simulink model "single_phase_converter_dq_i_pi_closeloop"  (R2022b)
settings: Solver=VariableStepAuto  StartTime=0.0  StopTime=0.1  FixedStep=1e-6  MaxStep=1e-8  RelTol=1e-7
model workspace (MAT data in the model file):
  Ts = 2.5e-05
  wr = 314.159265359
libraries: spsMosfetLib x4, spsSeriesRLCBranchLib x4, slpidlib x2, spsCurrentMeasurementLib x1, spsDCVoltageSourceLib x1, spsIdealSwitchLib x1, simulink x1, dspsigops x1, sps_lib x1
settings Model: Creator=SSC  LastModifiedBy=SSC

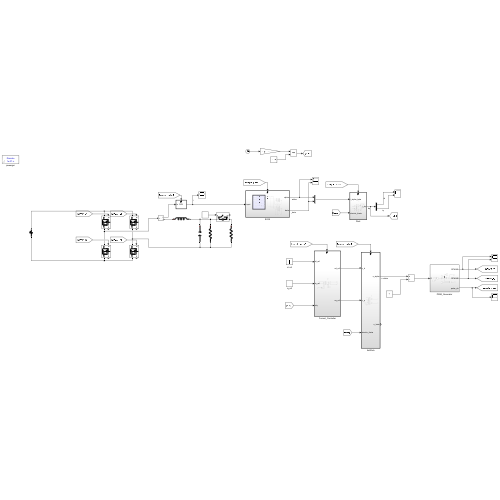
[thumbnail: Simulink's stored preview of the top-level diagram]
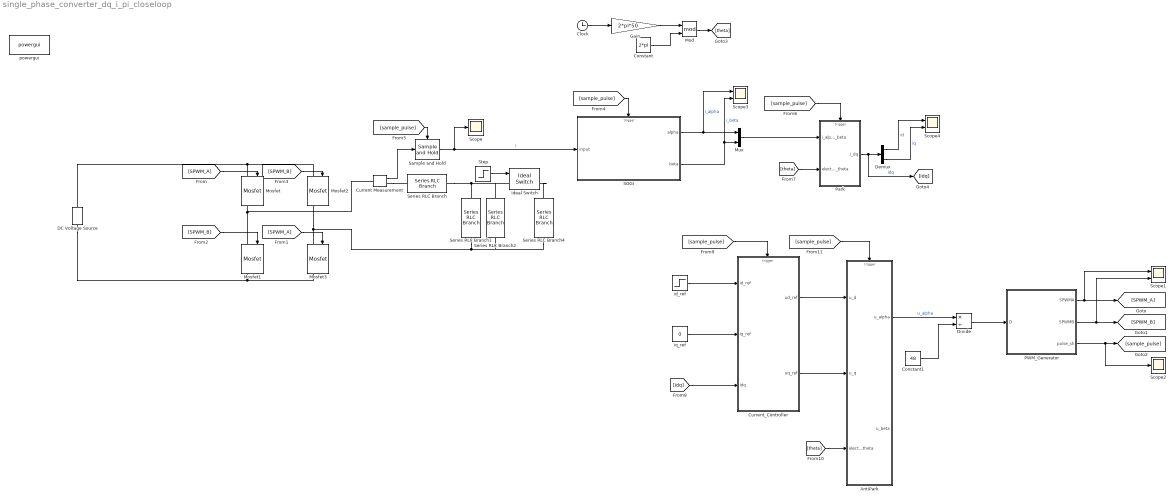
== system single_phase_converter_dq_i_pi_closeloop ==
  AntiPark : Subsystem
  Clock : Clock
  Constant : Constant  Value=2*pi
  Constant1 : Constant  Value=48
  Current Measurement : spsCurrentMeasurementLib/Current Measurement  PhasorSimulation=off  OutputType=Complex  PSBequivalent=0
  Current_Controller : Subsystem
  DC Voltage Source : spsDCVoltageSourceLib/DC Voltage Source  Amplitude=48  Measurements=None
  Demux : Demux  Outputs=2
  Divide : Product  Inputs=*/
  Gain : Gain  Gain=2*pi*50
  Ideal Switch : spsIdealSwitchLib/Ideal Switch  Ron=1e-5  Lon=0  IC=0  Rs=1e5  Cs=inf  Measurements=on
  Mod : Math  Operator=mod
  Mosfet{,1..3} (4 alike) : spsMosfetLib/Mosfet  Ron=0.1  Lon=0  Rd=0.01  Vfd=0  IC=0  Rs=1e5  Cs=inf  Measurements=on
  Mux : Mux  Inputs=2
  PWM_Generator : Subsystem
  Park : Subsystem
  SOGI : Subsystem  TreatAsAtomicUnit=on
  Sample and Hold : dspsigops/Sample and Hold  trig=Rising edge  initCond=0  latchinput=off
  Scope : Scope
  Scope1 : Scope  NumInputPorts=2
  Scope2 : Scope
  Scope3 : Scope  NumInputPorts=2
  Scope4 : Scope  NumInputPorts=2
  Series RLC Branch : spsSeriesRLCBranchLib/Series RLC Branch  LConnTagsString=__new0  RConnTagsString=__new0  BranchType=L  Resistance=1  Inductance=2e-3  SetiL0=off  InitialCurrent=0  Capacitance=1e-6  Setx0=off  InitialVoltage=0  Measurements=None
  Series RLC Branch1 : spsSeriesRLCBranchLib/Series RLC Branch  LConnTagsString=__new0  RConnTagsString=__new0  BranchType=C  Resistance=1  Inductance=1e-3  SetiL0=off  InitialCurrent=0  Capacitance=25e-6  Setx0=off  InitialVoltage=0  Measurements=None
  Series RLC Branch2 : spsSeriesRLCBranchLib/Series RLC Branch  LConnTagsString=__new0  RConnTagsString=__new0  BranchType=R  Resistance=12  Inductance=1e-3  SetiL0=off  InitialCurrent=0  Capacitance=1e-6  Setx0=off  InitialVoltage=0  Measurements=None
  Series RLC Branch4 : spsSeriesRLCBranchLib/Series RLC Branch  LConnTagsString=__new0  RConnTagsString=__new0  BranchType=R  Resistance=12  Inductance=1e-3  SetiL0=off  InitialCurrent=0  Capacitance=1e-6  Setx0=off  InitialVoltage=0  Measurements=None
  Step : Step  Time=0.1  SampleTime=0
  id_ref : Step  Time=0.05  Before=2  SampleTime=0
  iq_ref : Constant  Value=0
  powergui : sps_lib/powergui  Priority=1  SimulationMode=Discrete  SampleTime=1e-7  frequency=60  Iterations=50  frequencyindice=0  Pbase=100e6  ErrMax=1e-4  UnitsV=kV  UnitsW=MW  buscounter=0  FunctionMessages=off  echomessages=off  EnableUseOfTLC=off  CurrentSourceSwitches=off  DisableSnubberDevices=off  DisableRonSwitches=off  DisableVfSwitches=off  DisplayEquations=off  AutomaticDiscreteSolvers=off  SolverType=Tustin/Backward Euler (TBE)  Interpol=off  ExternalGateDelay=off  methode=off  Ts=100  x0status=blocks  SPID=on  SwTol=0  HookPort=off  NonlinearTolerance=1e-4  nMaxIteration=100  ContinueOnMaxIteration=off  RestoreLinks=warning  ResistiveCurrentMeasurement=off  Frange=[0:2:500]  Ylog=off  Xlog=on  ShowGrid=off  save=off  variable=ZData  structure=0  ZoomFFT=off  StartTime=0.0  cycles=1  DisplayStyle=1  fundamental=60  FreqAxis=off  MaxFrequency=1000  frequencyindicesteady=1  RmsSteady=1  display=off
  wires:
  Sample and Hold/1 -> SOGI/1(input), Scope/1  "i"
  [SPWM_A] -> Mosfet/1
  [SPWM_A] -> Mosfet3/1
  [SPWM_B] -> Mosfet1/1
  [SPWM_B] -> Mosfet2/1
  PWM_Generator/1(SPWMA) -> [SPWM_A], Scope1/1
  PWM_Generator/2(SPWMB) -> [SPWM_B], Scope1/2
  Divide/1 -> PWM_Generator/1(D)
  PWM_Generator/3(pulse_sh) -> Scope2/1, [sample_pulse]
  [sample_pulse] -> SOGI/Trigger
  Step/1 -> Ideal Switch/1
  Current Measurement/1 -> Sample and Hold/1
  [sample_pulse] -> Sample and Hold/Trigger
  SOGI/1(alpha) -> Mux/1, Scope3/1  "i_alpha"
  SOGI/2(beta) -> Mux/2, Scope3/2  "i_beta"
  Clock/1 -> Gain/1
  Gain/1 -> Mod/1
  Constant/1 -> Mod/2
  Mod/1 -> [theta]
  Mux/1 -> Park/1(i_alpha_beta)
  [sample_pulse] -> Park/Trigger
  [theta] -> Park/2(electric_theta)
  Park/1(i_dq) -> [idq], Demux/1  "idq"
  Demux/1 -> Scope4/1  "id"
  Demux/2 -> Scope4/2  "iq"
  iq_ref/1 -> Current_Controller/2(iq_ref)
  [idq] -> Current_Controller/3(idq)
  [sample_pulse] -> Current_Controller/Trigger
  Current_Controller/1(ud_ref) -> AntiPark/1(u_d)
  Current_Controller/2(uq_ref) -> AntiPark/2(u_q)
  [theta] -> AntiPark/3(electric_theta)
  [sample_pulse] -> AntiPark/Trigger
  AntiPark/1(u_alpha) -> Divide/1  "u_alpha"
  Constant1/1 -> Divide/2
  id_ref/1 -> Current_Controller/1(id_ref)
  connections:
  Series RLC Branch/RConn1 -- Series RLC Branch2/LConn1 -- Ideal Switch/LConn1 -- Series RLC Branch1/LConn1
  Mosfet1/LConn1 -- Current Measurement/LConn1 -- Mosfet/RConn1
  Mosfet/LConn1 -- Mosfet2/LConn1 -- DC Voltage Source/RConn1
  DC Voltage Source/LConn1 -- Mosfet3/RConn1 -- Mosfet1/RConn1
  Mosfet3/LConn1 -- Mosfet2/RConn1 -- Series RLC Branch2/RConn1 -- Series RLC Branch4/RConn1 -- Series RLC Branch1/RConn1
  Ideal Switch/RConn1 -- Series RLC Branch4/LConn1
  Current Measurement/RConn1 -- Series RLC Branch/LConn1

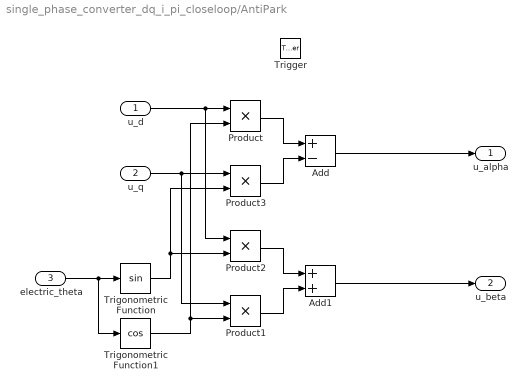
== system single_phase_converter_dq_i_pi_closeloop/AntiPark ==
  u_d : Inport
  u_q : Inport  Port=2
  electric_theta : Inport  Port=3
  Trigger : TriggerPort  VariantControl=(inherit)
  Add : Sum  Inputs=+-
  Add1 : Sum
  Product{,1..3} (4 alike) : Product
  Trigonometric Function : Trigonometry
  Trigonometric Function1 : Trigonometry  Operator=cos
  u_alpha : Outport
  u_beta : Outport  Port=2
  wires:
  electric_theta/1 -> Trigonometric Function1/1, Trigonometric Function/1
  u_d/1 -> Product2/1, Product/1
  Trigonometric Function1/1 -> Product/2, Product1/2
  u_q/1 -> Product1/1, Product3/1
  Trigonometric Function/1 -> Product2/2, Product3/2
  Product/1 -> Add/1
  Product3/1 -> Add/2
  Add/1 -> u_alpha/1
  Product2/1 -> Add1/1
  Product1/1 -> Add1/2
  Add1/1 -> u_beta/1

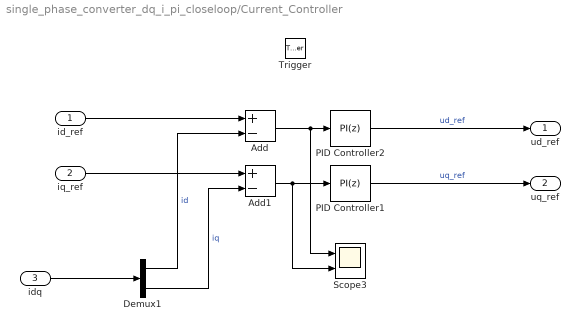
== system single_phase_converter_dq_i_pi_closeloop/Current_Controller ==
  id_ref : Inport
  iq_ref : Inport  Port=2
  idq : Inport  Port=3
  Trigger : TriggerPort  VariantControl=(inherit)
  Add : Sum  Inputs=+-
  Add1 : Sum  Inputs=+-
  Demux1 : Demux  Outputs=2
  PID Controller1 : slpidlib/PID Controller  Controller=PI  Form=Parallel  TimeDomain=Discrete-time  UseExternalTs=off  SampleTime=-1  IntegratorMethod=Trapezoidal  FilterMethod=Forward Euler  ControllerParametersSource=internal  P=1  I=1000  UseKiTs=off  D=0  N=100  UseFilter=on  TunerSelectOption=Transfer Function Based (PID Tuner App)  InitialConditionSource=internal  InitialConditionForIntegrator=0  InitialConditionForFilter=0  DifferentiatorICPrevScaledInput=0  ExternalReset=none  TrackingMode=off  Kt=1  LimitOutput=off  SatLimitsSource=internal  UpperSaturationLimit=inf  LowerSaturationLimit=-inf  LinearizeAsGain=on  AntiWindupMode=none  Kb=1  LimitIntegrator=off  UpperIntegratorSaturationLimit=inf  LowerIntegratorSaturationLimit=-inf  POutMin=[]  POutMax=[]  IOutMin=[]  IOutMax=[]  DOutMin=[]  DOutMax=[]  NOutMin=[]  NOutMax=[]  SumOutMin=[]  SumOutMax=[]  SaturationOutMin=[]  SaturationOutMax=[]  PParamMin=[]  PParamMax=[]  IParamMin=[]  IParamMax=[]  DParamMin=[]  DParamMax=[]  NParamMin=[]  NParamMax=[]  KbParamMin=[]  KbParamMax=[]  KtParamMin=[]  KtParamMax=[]  KbOutMin=[]  KbOutMax=[]  KtOutMin=[]  KtOutMax=[]  IntegratorOutMin=[]  IntegratorOutMax=[]  FilterOutMin=[]  FilterOutMax=[]  SumI1OutMin=[]  SumI1OutMax=[]  SumI2OutMin=[]  SumI2OutMax=[]  SumI3OutMin=[]  SumI3OutMax=[]  SumI4OutMin=[]  SumI4OutMax=[]  SumDOutMin=[]  SumDOutMax=[]  DifferentiatorOutMin=[]  DifferentiatorOutMax=[]  FilterDiffOutCoefMin=[]  FilterDiffOutCoefMax=[]  ReciprocalOutMin=[]  ReciprocalOutMax=[]  SumDenOutMin=[]  SumDenOutMax=[]  SumNumOutMin=[]  SumNumOutMax=[]  DivideOutMin=[]  DivideOutMax=[]  UdiffTsProdOutMin=[]  UdiffTsProdOutMax=[]  NTsProdOutMin=[]  NTsProdOutMax=[]  UintegralTsProdOutMin=[]  UintegralTsProdOutMax=[]  UngainTsProdOutMin=[]  UngainTsProdOutMax=[]  ClampingZeroOutDataTypeStr=Inherit: Inherit via back propagation  ClampingZeroOutMin=[]  ClampingZeroOutMax=[]  FilterDenConstantOutDataTypeStr=Inherit: Inherit via back propagation  FilterDenConstantOutMin=[]  FilterDenConstantOutMax=[]  PCopyOutDataTypeStr=Inherit: Inherit via back propagation  PCopyOutMin=[]  PCopyOutMax=[]  NCopyOutDataTypeStr=Inherit: Inherit via back propagation  NCopyOutMin=[]  NCopyOutMax=[]  IntegratorContinuousStateAttributes=''  IntegratorStateMustResolveToSignalObject=off  IntegratorRTWStateStorageClass=Auto  FilterContinuousStateAttributes=''  FilterStateMustResolveToSignalObject=off  FilterRTWStateStorageClass=Auto  ParallelPVariant=InternalParameters  IdealPVariant=Disabled  IVariant=InternalParameters  DVariant=Disabled  IntegratorVariant=Discrete  SatVariant=Disabled  AWVariant=Passthrough  PCopyVariant=Disabled  TRVariant=Disabled  FdbkBlocksVariant=Forward  IdealPFdbkVariant=Disabled  SatFdbkVariant=Disabled  DerivativeFilterVariant=Disabled  NVariant=Disabled  NCopyVariant=Disabled_SignalSpec  FilterICVariant=Disabled  IntegratorICVariant=InternalICs  ExternalResetVariant=Disabled  TRSumVariant=Passthrough  SumFdbkVariant=Disabled  SumVariant=Sum_PI  TsampFilterVariant=InternalTs  TsampNgainVariant=Passthrough  TsampIntegralVariant=Passthrough  ExternalSaturationOutDataTypeStr=Inherit: Same as second input
  PID Controller2 : slpidlib/PID Controller  Controller=PI  Form=Parallel  TimeDomain=Discrete-time  UseExternalTs=off  SampleTime=-1  IntegratorMethod=Trapezoidal  FilterMethod=Forward Euler  ControllerParametersSource=internal  P=10  I=1000  UseKiTs=off  D=0  N=100  UseFilter=on  TunerSelectOption=Transfer Function Based (PID Tuner App)  InitialConditionSource=internal  InitialConditionForIntegrator=0  InitialConditionForFilter=0  DifferentiatorICPrevScaledInput=0  ExternalReset=none  TrackingMode=off  Kt=1  LimitOutput=off  SatLimitsSource=internal  UpperSaturationLimit=inf  LowerSaturationLimit=-inf  LinearizeAsGain=on  AntiWindupMode=none  Kb=1  LimitIntegrator=off  UpperIntegratorSaturationLimit=inf  LowerIntegratorSaturationLimit=-inf  POutMin=[]  POutMax=[]  IOutMin=[]  IOutMax=[]  DOutMin=[]  DOutMax=[]  NOutMin=[]  NOutMax=[]  SumOutMin=[]  SumOutMax=[]  SaturationOutMin=[]  SaturationOutMax=[]  PParamMin=[]  PParamMax=[]  IParamMin=[]  IParamMax=[]  DParamMin=[]  DParamMax=[]  NParamMin=[]  NParamMax=[]  KbParamMin=[]  KbParamMax=[]  KtParamMin=[]  KtParamMax=[]  KbOutMin=[]  KbOutMax=[]  KtOutMin=[]  KtOutMax=[]  IntegratorOutMin=[]  IntegratorOutMax=[]  FilterOutMin=[]  FilterOutMax=[]  SumI1OutMin=[]  SumI1OutMax=[]  SumI2OutMin=[]  SumI2OutMax=[]  SumI3OutMin=[]  SumI3OutMax=[]  SumI4OutMin=[]  SumI4OutMax=[]  SumDOutMin=[]  SumDOutMax=[]  DifferentiatorOutMin=[]  DifferentiatorOutMax=[]  FilterDiffOutCoefMin=[]  FilterDiffOutCoefMax=[]  ReciprocalOutMin=[]  ReciprocalOutMax=[]  SumDenOutMin=[]  SumDenOutMax=[]  SumNumOutMin=[]  SumNumOutMax=[]  DivideOutMin=[]  DivideOutMax=[]  UdiffTsProdOutMin=[]  UdiffTsProdOutMax=[]  NTsProdOutMin=[]  NTsProdOutMax=[]  UintegralTsProdOutMin=[]  UintegralTsProdOutMax=[]  UngainTsProdOutMin=[]  UngainTsProdOutMax=[]  ClampingZeroOutDataTypeStr=Inherit: Inherit via back propagation  ClampingZeroOutMin=[]  ClampingZeroOutMax=[]  FilterDenConstantOutDataTypeStr=Inherit: Inherit via back propagation  FilterDenConstantOutMin=[]  FilterDenConstantOutMax=[]  PCopyOutDataTypeStr=Inherit: Inherit via back propagation  PCopyOutMin=[]  PCopyOutMax=[]  NCopyOutDataTypeStr=Inherit: Inherit via back propagation  NCopyOutMin=[]  NCopyOutMax=[]  IntegratorContinuousStateAttributes=''  IntegratorStateMustResolveToSignalObject=off  IntegratorRTWStateStorageClass=Auto  FilterContinuousStateAttributes=''  FilterStateMustResolveToSignalObject=off  FilterRTWStateStorageClass=Auto  ParallelPVariant=InternalParameters  IdealPVariant=Disabled  IVariant=InternalParameters  DVariant=Disabled  IntegratorVariant=Discrete  SatVariant=Disabled  AWVariant=Passthrough  PCopyVariant=Disabled  TRVariant=Disabled  FdbkBlocksVariant=Forward  IdealPFdbkVariant=Disabled  SatFdbkVariant=Disabled  DerivativeFilterVariant=Disabled  NVariant=Disabled  NCopyVariant=Disabled_SignalSpec  FilterICVariant=Disabled  IntegratorICVariant=InternalICs  ExternalResetVariant=Disabled  TRSumVariant=Passthrough  SumFdbkVariant=Disabled  SumVariant=Sum_PI  TsampFilterVariant=InternalTs  TsampNgainVariant=Passthrough  TsampIntegralVariant=Passthrough  ExternalSaturationOutDataTypeStr=Inherit: Same as second input
  Scope3 : Scope  NumInputPorts=2
  ud_ref : Outport
  uq_ref : Outport  Port=2
  wires:
  Demux1/2 -> Add1/2  "iq"
  id_ref/1 -> Add/1
  Add1/1 -> Scope3/2, PID Controller1/1
  Demux1/1 -> Add/2  "id"
  iq_ref/1 -> Add1/1
  Add/1 -> Scope3/1, PID Controller2/1
  idq/1 -> Demux1/1
  PID Controller2/1 -> ud_ref/1  "ud_ref"
  PID Controller1/1 -> uq_ref/1  "uq_ref"

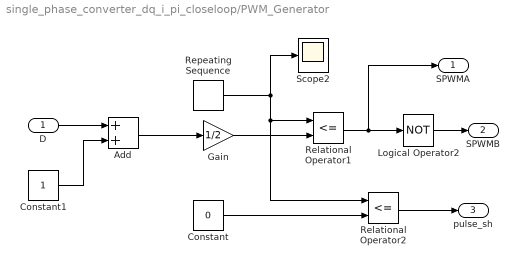
== system single_phase_converter_dq_i_pi_closeloop/PWM_Generator ==
  D : Inport
  Add : Sum
  Constant : Constant  Value=0
  Constant1 : Constant
  Gain : Gain  Gain=1/2
  Logical Operator2 : Logic  Operator=NOT  AllPortsSameDT=off  OutDataTypeStr=boolean
  Relational Operator1 : RelationalOperator  Operator=<=  OutDataTypeStr=boolean  RndMeth=Simplest  InputSameDT=off
  Relational Operator2 : RelationalOperator  Operator=<=  OutDataTypeStr=boolean  RndMeth=Simplest  InputSameDT=off
  Repeating Sequence : simulink/Sources/Repeating Sequence  rep_seq_t=[0 0.125e-4 0.25e-4]  rep_seq_y=[0 1 0]
  Scope2 : Scope
  SPWMA : Outport
  SPWMB : Outport  Port=2
  pulse_sh : Outport  Port=3
  wires:
  Relational Operator1/1 -> SPWMA/1, Logical Operator2/1
  Logical Operator2/1 -> SPWMB/1
  Repeating Sequence/1 -> Relational Operator2/1, Relational Operator1/1, Scope2/1
  Relational Operator2/1 -> pulse_sh/1
  Constant/1 -> Relational Operator2/2
  Add/1 -> Gain/1
  D/1 -> Add/1
  Gain/1 -> Relational Operator1/2
  Constant1/1 -> Add/2

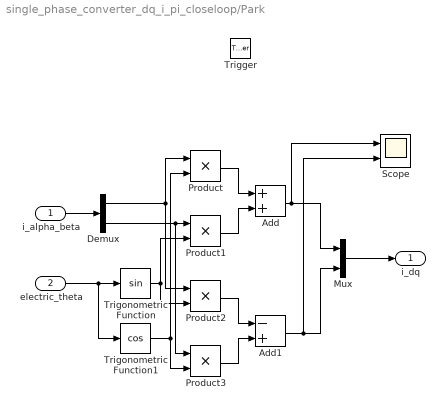
== system single_phase_converter_dq_i_pi_closeloop/Park ==
  i_alpha_beta : Inport
  electric_theta : Inport  Port=2
  Trigger : TriggerPort  VariantControl=(inherit)
  Add : Sum
  Add1 : Sum  Inputs=-+
  Demux : Demux  Outputs=2
  Mux : Mux  Inputs=2
  Product{,1..3} (4 alike) : Product
  Scope : Scope  NumInputPorts=2
  Trigonometric Function : Trigonometry
  Trigonometric Function1 : Trigonometry  Operator=cos
  i_dq : Outport
  wires:
  electric_theta/1 -> Trigonometric Function1/1, Trigonometric Function/1
  Trigonometric Function1/1 -> Product3/2, Product/2
  Demux/2 -> Product3/1, Product1/1
  Trigonometric Function/1 -> Product2/2, Product1/2
  Product/1 -> Add/1
  Product1/1 -> Add/2
  Product2/1 -> Add1/1
  Product3/1 -> Add1/2
  Add/1 -> Scope/1, Mux/1
  Add1/1 -> Scope/2, Mux/2
  Demux/1 -> Product/1, Product2/1
  i_alpha_beta/1 -> Demux/1
  Mux/1 -> i_dq/1

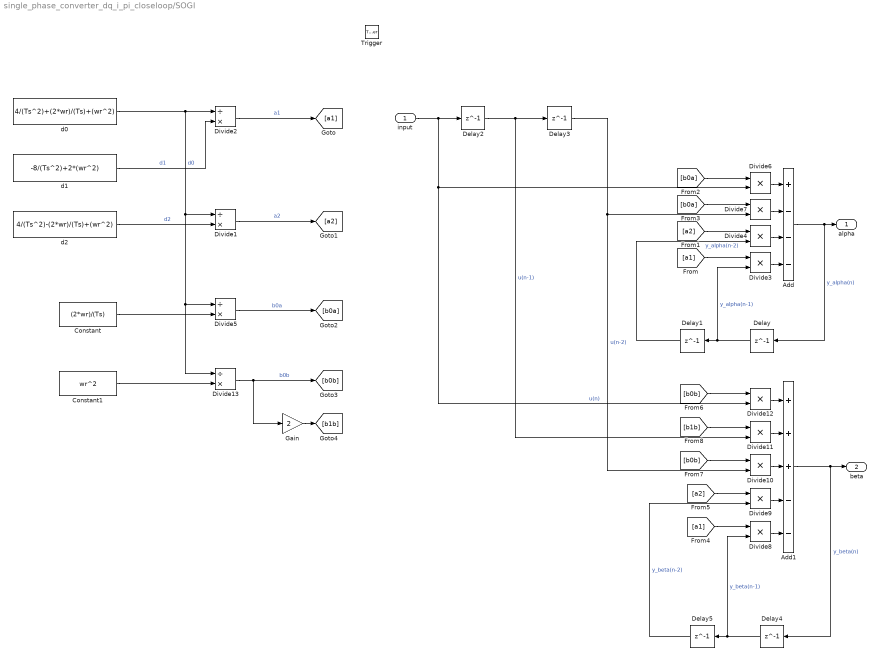
== system single_phase_converter_dq_i_pi_closeloop/SOGI ==
  input : Inport
  Trigger : TriggerPort  VariantControl=(inherit)
  Add : Sum  Inputs=+---
  Add1 : Sum  Inputs=+++--
  Constant : Constant  Value=(2*wr)/(Ts)
  Constant1 : Constant  Value=wr^2
  Delay{,1..5} (6 alike) : Delay  DelayLength=1  InitialCondition=0
  Divide{1..2,5,13} (4 alike) : Product  Inputs=/*
  Divide{3..4,6..12} (9 alike) : Product  Inputs=**
  Gain : Gain  Gain=2
  d0 : Constant  Value=4/(Ts^2)+(2*wr)/(Ts)+(wr^2)
  d1 : Constant  Value=-8/(Ts^2)+2*(wr^2)
  d2 : Constant  Value=4/(Ts^2)-(2*wr)/(Ts)+(wr^2)
  alpha : Outport
  beta : Outport  Port=2
  wires:
  d0/1 -> Divide2/1, Divide5/1, Divide13/1, Divide1/1  "d0"
  d1/1 -> Divide2/2  "d1"
  d2/1 -> Divide1/2  "d2"
  Divide2/1 -> [a1]  "a1"
  Divide1/1 -> [a2]  "a2"
  Add/1 -> Delay/1, alpha/1  "y_alpha(n)"
  Delay/1 -> Divide3/2, Delay1/1  "y_alpha(n-1)"
  Delay1/1 -> Divide4/2  "y_alpha(n-2)"
  Divide3/1 -> Add/4
  [a1] -> Divide3/1
  Divide4/1 -> Add/3
  [a2] -> Divide4/1
  Divide5/1 -> [b0a]  "b0a"
  Constant/1 -> Divide5/2
  Divide6/1 -> Add/1
  [b0a] -> Divide6/1
  Divide7/1 -> Add/2
  input/1 -> Divide12/2, Divide6/2, Delay2/1  "u(n)"
  Delay2/1 -> Divide11/2, Delay3/1  "u(n-1)"
  Delay3/1 -> Divide10/2, Divide7/2  "u(n-2)"
  [b0a] -> Divide7/1
  Add1/1 -> Delay4/1, beta/1  "y_beta(n)"
  Delay5/1 -> Divide9/2  "y_beta(n-2)"
  Delay4/1 -> Divide8/2, Delay5/1  "y_beta(n-1)"
  Divide8/1 -> Add1/5
  [a1] -> Divide8/1
  Divide9/1 -> Add1/4
  [a2] -> Divide9/1
  Divide10/1 -> Add1/3
  Divide11/1 -> Add1/2
  Divide12/1 -> Add1/1
  Constant1/1 -> Divide13/2
  Divide13/1 -> Gain/1, [b0b]  "b0b"
  Gain/1 -> [b1b]
  [b0b] -> Divide12/1
  [b0b] -> Divide10/1
  [b1b] -> Divide11/1
